simulink model "eVTOL_System"  (R2024b)
settings: Solver=FixedStepAuto  StartTime=0.0  StopTime=inf  RelTol=1e-3
undefined symbols (not defined in the file): airspeed, Battery, BCE12, BCE_Set_init, BMS_Controller_State, C, Cell10_P, Cell11_P, Cell12_P, Cell13_P, Cell14_P, Cell15_P, Cell16_P, Cell17_P, Cell18_P, Cell19_P, Cell1_N, Cell1_P, Cell20_P, Cell21_P, Cell22_P, Cell23_P, Cell24_P, Cell2_P, Cell3_P, Cell4_P, Cell5_P, Cell6_P, Cell7_P, Cell8_P, Cell9_P, Charging_State, CityMission, control, controlParams, ControlSampleTime, CriticalTiltAngle, currentFactor, CV_Gain, ddx, ddy, ddz, Device_01, Device_02, DiscIntNeverNeededParam, dx, dy, dz, Earth, env, F, F28379D_ADC_MaxCount, F28379D_ADC_Vmax, FixedWingMission, flightState, Foc_Ki_IxTcpu, Foc_Ki_S, Foc_Kp_I, Foc_Kp_S, fractalcoef ... (+68)
libraries: fl_lib x1115, nesl_utility x617, slrealtimeethercatlib x217, simulink x130, canmsglib x101, speedgoatlib_IO611_obsolete x91, slpidlib x49, mcbcontrolslib x44, slrealtimeutilitieslib x35, speedgoatlib_hdlCoder_IO3xx x31, dspstat3 x24, mcbpositiondecoderlib x12
(part 6 of 31)

== system eVTOL_System/Battery System/Battery/Battery Pack/100-Cell ==
  Ambient_Temperature : Inport
  Controlled Temperature Source : fl_lib/Thermal/Thermal Sources/Controlled Temperature Source
      settings: LibrarySourceBlock=|
      | BatteryPack_lib/CellModule1TC/Controlled
      | Temperature Source
  Delay : Delay
  Delay1 : Delay
  Delay2 : Delay
  Faults : Subsystem
  Faults1 : Subsystem
  Faults2 : Subsystem
  Module3 : BatteryModuleLibrary96v_lib/Module1  BatteryCapacityCell=100 A*hr  ExtrapolationMethodCell=simscape.enum.extrapolation.nearest  SOCBreakpointsCell=[0, .1, .25, .5, .75, .9, 1]  TemperatureBreakpointsCell=[278, 293, 313] K  OpenCircuitVoltageThermalCell=[3.49, 3.5, 3.51; 3.55, 3.57, 3.56; 3.62, 3.63, 3.64; 3.71, 3.71, 3.72; 3.91, 3.93, 3.94; 4.07, 4.08, 4.08; 4.19, 4.19, 4.19] V  VoltageRangeCell=[0, inf] V  ResistanceSOCBreakpointsCell=[0, .1, .25, .5, .75, .9, 1]  ResistanceTemperatureBreakpointsCell=[278, 293, 313] K  R0ThermalCell=[.00117, .00085, .0009; .0011, .00085, .0009; .00114, .00087, .00092; .00107, .00082, .00088; .00107, .00083, .00091; .00113, .00085, .00089; .00116, .00085, .00089] Ohm  BatteryThermalMassCell=1000 J/K  AmbientResistance=25 K/W  P=1  S=24  socCell_specify=off  socCell_priority=High  socCell=repmat(1, 24, 1)  socCell_nominal_specify=off  socCell_nominal_value=1  socCell_nominal_unit=1  numCycles_specify=off  numCycles_priority=High  numCycles=repmat(0, 24, 1)  numCycles_nominal_specify=off  numCycles_nominal_value=1  numCycles_nominal_unit=1  batteryVoltage_specify=off  batteryVoltage_priority=None  batteryVoltage=repmat(0, 24, 1) V  batteryVoltage_nominal_specify=off  batteryVoltage_nominal_value=1  batteryVoltage_nominal_unit=V  batteryCurrent_specify=off  batteryCurrent_priority=None  batteryCurrent=repmat(0, 24, 1) A  batteryCurrent_nominal_specify=off  batteryCurrent_nominal_value=1  batteryCurrent_nominal_unit=A  batteryTemperature_specify=off  batteryTemperature_priority=High  batteryTemperature=repmat(298.15, 24, 1) K  batteryTemperature_nominal_specify=off  batteryTemperature_nominal_value=1  batteryTemperature_nominal_unit=K  vParallelAssembly_specify=off  vParallelAssembly_priority=None  vParallelAssembly=repmat(0, 24, 1) V  vParallelAssembly_nominal_specify=off  vParallelAssembly_nominal_value=1  vParallelAssembly_nominal_unit=V  socParallelAssembly_specify=off  socParallelAssembly_priority=None  socParallelAssembly=repmat(1, 24, 1)  socParallelAssembly_nominal_specify=off  socParallelAssembly_nominal_value=1  socParallelAssembly_nominal_unit=1
      settings: InternalSimscapePortConfiguration="{\"Bottom\":[{\"id\":\"n\",\"label\":\"-\",\"type\":\"foundation.electrical.electrical\"}],\"Left\":[{\"id\":\"AmbH\",\"label\":\"AmbH\",\"type\":\"foundation.thermal.thermal\"}],\"Right\":[{\"id\":\"PositiveBus\",\"label\":\"+Bus\",\"type\":\"foundation.electrical.electrical\"},{\"id\":\"NegativeBus\",\"label\":\"-Bus\",\"type\":\"foundation.electrical.electrical\"}],\"Top\":[{\"id\":\"p\",\"label\":\"+\",\"type\":\"foundation.electrical.electrical\"}]}"
  Module4 : BatteryModuleLibrary150V_lib/Module1  BatteryCapacityCell=100 A*hr  ExtrapolationMethodCell=simscape.enum.extrapolation.nearest  SOCBreakpointsCell=[0, .1, .25, .5, .75, .9, 1]  TemperatureBreakpointsCell=[278, 293, 313] K  OpenCircuitVoltageThermalCell=[3.49, 3.5, 3.51; 3.55, 3.57, 3.56; 3.62, 3.63, 3.64; 3.71, 3.71, 3.72; 3.91, 3.93, 3.94; 4.07, 4.08, 4.08; 4.19, 4.19, 4.19] V  VoltageRangeCell=[0, inf] V  ResistanceSOCBreakpointsCell=[0, .1, .25, .5, .75, .9, 1]  ResistanceTemperatureBreakpointsCell=[278, 293, 313] K  R0ThermalCell=[.00117, .00085, .0009; .0011, .00085, .0009; .00114, .00087, .00092; .00107, .00082, .00088; .00107, .00083, .00091; .00113, .00085, .00089; .00116, .00085, .00089] Ohm  BatteryThermalMassCell=1000 J/K  AmbientResistance=25 K/W  P=1  S=38  socCell_specify=off  socCell_priority=High  socCell=repmat(1, 38, 1)  socCell_nominal_specify=off  socCell_nominal_value=1  socCell_nominal_unit=1  numCycles_specify=off  numCycles_priority=High  numCycles=repmat(0, 38, 1)  numCycles_nominal_specify=off  numCycles_nominal_value=1  numCycles_nominal_unit=1  batteryVoltage_specify=off  batteryVoltage_priority=None  batteryVoltage=repmat(0, 38, 1) V  batteryVoltage_nominal_specify=off  batteryVoltage_nominal_value=1  batteryVoltage_nominal_unit=V  batteryCurrent_specify=off  batteryCurrent_priority=None  batteryCurrent=repmat(0, 38, 1) A  batteryCurrent_nominal_specify=off  batteryCurrent_nominal_value=1  batteryCurrent_nominal_unit=A  batteryTemperature_specify=off  batteryTemperature_priority=High  batteryTemperature=repmat(298.15, 38, 1) K  batteryTemperature_nominal_specify=off  batteryTemperature_nominal_value=1  batteryTemperature_nominal_unit=K  vParallelAssembly_specify=off  vParallelAssembly_priority=None  vParallelAssembly=repmat(0, 38, 1) V  vParallelAssembly_nominal_specify=off  vParallelAssembly_nominal_value=1  vParallelAssembly_nominal_unit=V  socParallelAssembly_specify=off  socParallelAssembly_priority=None  socParallelAssembly=repmat(1, 38, 1)  socParallelAssembly_nominal_specify=off  socParallelAssembly_nominal_value=1  socParallelAssembly_nominal_unit=1
      settings: InternalSimscapePortConfiguration="{\"Bottom\":[{\"id\":\"n\",\"label\":\"-\",\"type\":\"foundation.electrical.electrical\"}],\"Left\":[{\"id\":\"AmbH\",\"label\":\"AmbH\",\"type\":\"foundation.thermal.thermal\"}],\"Right\":[{\"id\":\"PositiveBus\",\"label\":\"+Bus\",\"type\":\"foundation.electrical.electrical\"},{\"id\":\"NegativeBus\",\"label\":\"-Bus\",\"type\":\"foundation.electrical.electrical\"}],\"Top\":[{\"id\":\"p\",\"label\":\"+\",\"type\":\"foundation.electrical.electrical\"}]}"
  Module5 : BatteryModuleLibrary150V_lib/Module1  BatteryCapacityCell=100 A*hr  ExtrapolationMethodCell=simscape.enum.extrapolation.nearest  SOCBreakpointsCell=[0, .1, .25, .5, .75, .9, 1]  TemperatureBreakpointsCell=[278, 293, 313] K  OpenCircuitVoltageThermalCell=[3.49, 3.5, 3.51; 3.55, 3.57, 3.56; 3.62, 3.63, 3.64; 3.71, 3.71, 3.72; 3.91, 3.93, 3.94; 4.07, 4.08, 4.08; 4.19, 4.19, 4.19] V  VoltageRangeCell=[0, inf] V  ResistanceSOCBreakpointsCell=[0, .1, .25, .5, .75, .9, 1]  ResistanceTemperatureBreakpointsCell=[278, 293, 313] K  R0ThermalCell=[.00117, .00085, .0009; .0011, .00085, .0009; .00114, .00087, .00092; .00107, .00082, .00088; .00107, .00083, .00091; .00113, .00085, .00089; .00116, .00085, .00089] Ohm  BatteryThermalMassCell=1000 J/K  AmbientResistance=25 K/W  P=1  S=38  socCell_specify=off  socCell_priority=High  socCell=repmat(1, 38, 1)  socCell_nominal_specify=off  socCell_nominal_value=1  socCell_nominal_unit=1  numCycles_specify=off  numCycles_priority=High  numCycles=repmat(0, 38, 1)  numCycles_nominal_specify=off  numCycles_nominal_value=1  numCycles_nominal_unit=1  batteryVoltage_specify=off  batteryVoltage_priority=None  batteryVoltage=repmat(0, 38, 1) V  batteryVoltage_nominal_specify=off  batteryVoltage_nominal_value=1  batteryVoltage_nominal_unit=V  batteryCurrent_specify=off  batteryCurrent_priority=None  batteryCurrent=repmat(0, 38, 1) A  batteryCurrent_nominal_specify=off  batteryCurrent_nominal_value=1  batteryCurrent_nominal_unit=A  batteryTemperature_specify=off  batteryTemperature_priority=High  batteryTemperature=repmat(298.15, 38, 1) K  batteryTemperature_nominal_specify=off  batteryTemperature_nominal_value=1  batteryTemperature_nominal_unit=K  vParallelAssembly_specify=off  vParallelAssembly_priority=None  vParallelAssembly=repmat(0, 38, 1) V  vParallelAssembly_nominal_specify=off  vParallelAssembly_nominal_value=1  vParallelAssembly_nominal_unit=V  socParallelAssembly_specify=off  socParallelAssembly_priority=None  socParallelAssembly=repmat(1, 38, 1)  socParallelAssembly_nominal_specify=off  socParallelAssembly_nominal_value=1  socParallelAssembly_nominal_unit=1
      settings: InternalSimscapePortConfiguration="{\"Bottom\":[{\"id\":\"n\",\"label\":\"-\",\"type\":\"foundation.electrical.electrical\"}],\"Left\":[{\"id\":\"AmbH\",\"label\":\"AmbH\",\"type\":\"foundation.thermal.thermal\"}],\"Right\":[{\"id\":\"PositiveBus\",\"label\":\"+Bus\",\"type\":\"foundation.electrical.electrical\"},{\"id\":\"NegativeBus\",\"label\":\"-Bus\",\"type\":\"foundation.electrical.electrical\"}],\"Top\":[{\"id\":\"p\",\"label\":\"+\",\"type\":\"foundation.electrical.electrical\"}]}"
  Mux : Mux  Inputs=3
  Mux1 : Mux  Inputs=3
  Mux2 : Mux  Inputs=3
  PS-Simulink Converter{,1..2,5..6} (5 alike) : nesl_utility/PS-Simulink Converter  PhysicalDomain=network_engine_domain  SubClassName=ps_output  LeftPortType=input  RightPortType=output  PseudoPeriodic=off  Frequencies=[]  VectorFormat=inherit  Unit=inherit  AffineConversion=off
  Passive Balancing Interface : batt_lib/HIL/Passive Balancing Interface  balancingCircuitCount=24
      settings: InternalSimscapePortConfiguration="{\"Bottom\":[],\"Left\":[{\"id\":\"PositiveBus\",\"label\":\"+\",\"type\":\"foundation.electrical.electrical\"},{\"id\":\"NegativeBus\",\"label\":\"-\",\"type\":\"foundation.electrical.electrical\"}],\"Right\":[{\"id\":\"balancingCurrent\",\"label\":\"Ibat\",\"type\":\"input\"},{\"id\":\"balancingVoltage\",\"label\":\"Vbat\",\"type\":\"output\"}],\"Top\":[]}"
  Passive Balancing Interface1 : batt_lib/HIL/Passive Balancing Interface  balancingCircuitCount=38
      settings: InternalSimscapePortConfiguration="{\"Bottom\":[],\"Left\":[{\"id\":\"PositiveBus\",\"label\":\"+\",\"type\":\"foundation.electrical.electrical\"},{\"id\":\"NegativeBus\",\"label\":\"-\",\"type\":\"foundation.electrical.electrical\"}],\"Right\":[{\"id\":\"balancingCurrent\",\"label\":\"Ibat\",\"type\":\"input\"},{\"id\":\"balancingVoltage\",\"label\":\"Vbat\",\"type\":\"output\"}],\"Top\":[]}"
  Passive Balancing Interface2 : batt_lib/HIL/Passive Balancing Interface  balancingCircuitCount=38
      settings: InternalSimscapePortConfiguration="{\"Bottom\":[],\"Left\":[{\"id\":\"PositiveBus\",\"label\":\"+\",\"type\":\"foundation.electrical.electrical\"},{\"id\":\"NegativeBus\",\"label\":\"-\",\"type\":\"foundation.electrical.electrical\"}],\"Right\":[{\"id\":\"balancingCurrent\",\"label\":\"Ibat\",\"type\":\"input\"},{\"id\":\"balancingVoltage\",\"label\":\"Vbat\",\"type\":\"output\"}],\"Top\":[]}"
  Probe : SimscapeProbe  BoundBlock=16864  Variables={batteryTemperature, batteryVoltage, socParallelAssembly}
  Probe1 : SimscapeProbe  BoundBlock=17225  Variables={batteryTemperature, batteryVoltage, socParallelAssembly}
  Probe2 : SimscapeProbe  BoundBlock=17226  Variables={batteryTemperature, batteryVoltage, socParallelAssembly}
  Simulink-PS Converter{,1..3} (4 alike) : nesl_utility/Simulink-PS Converter  PhysicalDomain=network_engine_domain  SubClassName=ps_input  LeftPortType=input  RightPortType=output  PseudoPeriodic=off  Frequencies=[]  NoiseDistribution=none  NoiseParameters=[]  Unit=1  AffineConversion=off  FilteringAndDerivatives=provide  SimscapeFilterOrder=1  InputFilterTimeConstant=0.001  UdotUserProvided=0
      Simulink-PS Converter1 settings: LibrarySourceBlock=|
      | BatteryPack_lib/CellModule1TC/Simulink-PS
      | Converter1
  Terminator : Terminator
  Terminator1 : Terminator
  Terminator2 : Terminator
  Trigger_Faults : Subsystem
  Voltage Sensor : fl_lib/Electrical/Electrical Sensors/Voltage Sensor
  Voltage Sensor1 : fl_lib/Electrical/Electrical Sensors/Voltage Sensor
  Batt+ : PMIOPort  Side=Right
  Batt- : PMIOPort  Port=2  Side=Right
  Cells : PMIOPort  Port=3  Side=Right
  Cells1 : PMIOPort  Port=4  Side=Right
  Cells2 : PMIOPort  Port=5  Side=Right
  Cell_Voltages : Outport
  Cell_Temperatures : Outport  Port=2
  Cell_SOCs : Outport  Port=3
  tag scope: Cell_Voltages1=global, Cell_Voltages2=global, Pack_Voltage_24Cells=global, Pack_Voltage_76Cells=global
  wires:
  [Balancing_Currents] -> Delay/1
  Delay/1 -> Simulink-PS Converter/1
  Ambient_Temperature/1 -> Simulink-PS Converter1/1
  [Balancing_Currents1] -> Delay1/1
  Delay1/1 -> Simulink-PS Converter2/1
  [Balancing_Currents2] -> Delay2/1
  Delay2/1 -> Simulink-PS Converter3/1
  Mux1/1 -> Cell_Voltages/1
  Mux/1 -> Cell_Temperatures/1
  Mux2/1 -> Cell_SOCs/1
  Probe1/2 -> [Cell_Voltages1], [Vol2]
  Probe/1 -> [Temp1]
  Probe/2 -> [Vol1]
  Probe/3 -> [soc1]
  Probe1/1 -> [Temp2]
  Probe1/3 -> [soc2]
  Probe2/1 -> [Temp3]
  Probe2/2 -> [Cell_Voltages2], [Vol3]
  Probe2/3 -> [soc3]
  [Vol1] -> Mux1/1
  [Vol2] -> Mux1/2
  [Vol3] -> Mux1/3
  [Temp1] -> Mux/1
  [Temp2] -> Mux/2
  [Temp3] -> Mux/3
  [soc1] -> Mux2/1
  [soc2] -> Mux2/2
  [soc3] -> Mux2/3
  PS-Simulink Converter5/1 -> [Pack_Voltage_76Cells]
  PS-Simulink Converter6/1 -> [Pack_Voltage_24Cells]
  PS-Simulink Converter/1 -> Terminator/1
  Trigger_Faults/1(ShortCircuit) -> Faults/1(Short_Circuits), Faults2/1(Short_Circuits), Faults1/1(Short_Circuits)
  PS-Simulink Converter1/1 -> Terminator1/1
  PS-Simulink Converter2/1 -> Terminator2/1
  connections:
  Module3/LConn1 -- Module4/LConn1 -- Module5/LConn1 -- Controlled Temperature Source/LConn1
  Passive Balancing Interface/LConn1 -- Module3/RConn1 -- Faults/RConn1
  Passive Balancing Interface/RConn1 -- Simulink-PS Converter/RConn1
  PS-Simulink Converter/LConn1 -- Passive Balancing Interface/RConn2
  Passive Balancing Interface/LConn2 -- Module3/RConn2 -- Faults/RConn3
  Cells/RConn1 -- Faults/RConn2
  Simulink-PS Converter1/RConn1 -- Controlled Temperature Source/RConn1
  Module5/LConn2 -- Voltage Sensor1/LConn1 -- Voltage Sensor/RConn2 -- Module3/RConn3
  Batt-/RConn1 -- Voltage Sensor1/RConn2 -- Module4/RConn3
  Module4/LConn2 -- Module5/RConn3
  Faults1/RConn3 -- Module5/RConn2 -- Passive Balancing Interface1/LConn2
  Faults1/RConn1 -- Module5/RConn1 -- Passive Balancing Interface1/LConn1
  Passive Balancing Interface1/RConn1 -- Simulink-PS Converter2/RConn1
  Cells1/RConn1 -- Faults1/RConn2
  PS-Simulink Converter1/LConn1 -- Passive Balancing Interface1/RConn2
  Passive Balancing Interface2/LConn2 -- Faults2/RConn3 -- Module4/RConn2
  Passive Balancing Interface2/LConn1 -- Faults2/RConn1 -- Module4/RConn1
  Passive Balancing Interface2/RConn1 -- Simulink-PS Converter3/RConn1
  Faults2/RConn2 -- Cells2/RConn1
  PS-Simulink Converter2/LConn1 -- Passive Balancing Interface2/RConn2
  PS-Simulink Converter5/LConn1 -- Voltage Sensor1/RConn1
  PS-Simulink Converter6/LConn1 -- Voltage Sensor/RConn1
  Batt+/RConn1 -- Voltage Sensor/LConn1 -- Module3/LConn2

== system eVTOL_System/Battery System/Battery/HW Interface/BCE - HIL ==
  Sensor_Values_Sim : Inport
  Add : Sum  Inputs=+
  Add1 : Sum  Inputs=+
  Add2 : Sum  Inputs=+
  Battery Cell Emulator : Subsystem
  Bus Creator : BusCreator  Inputs=6
  Data Type Conversion : DataTypeConversion  SaturateOnIntegerOverflow=off  RndMeth=Floor
  Selector1 : Subsystem
  Shunt Emulator : Subsystem
  Temperature Emulator : Subsystem
  Cells_IN : PMIOPort  Side=Left
  Cells_OUT : PMIOPort  Port=2  Side=Right
  Sensor_Values_Real : Outport
  tag scope: Balancing_Currents=global
  wires:
  Sensor_Values_Sim/1 -> Battery Cell Emulator/1(Sensor_Values_Sim), Shunt Emulator/1(Sensor_Values_Sim), Temperature Emulator/1(Sensor_Values_Sim)
  Battery Cell Emulator/2(Cell_Voltages) -> Add1/1, Selector1/1(24Cells)
  Temperature Emulator/1(Cell_Temperatures) -> Bus Creator/2  "Cell_Temperatures"
  Add/1 -> Bus Creator/3  "Pack_Voltage"
  Bus Creator/1 -> Sensor_Values_Real/1
  Battery Cell Emulator/1(Current_Values) -> Data Type Conversion/1
  Data Type Conversion/1 -> [Balancing_Currents]
  Selector1/1(100Cells) -> Bus Creator/1, Add/1  "Cell_Voltages"
  Battery Cell Emulator/3(OtherVoltages) -> Add2/1, Selector1/2(76Cells)
  Add1/1 -> Bus Creator/4  "Pack_Voltage1"
  Add2/1 -> Bus Creator/5  "Pack_Voltage2"
  Shunt Emulator/1(Pack_Current) -> Bus Creator/6  "Pack_Current"
  connections:
  Cells_OUT/RConn1 -- Cells_IN/RConn1

== system eVTOL_System/Battery System/Battery/HW Interface/MIL ==
  Sensor_Values_Sim : Inport
  Cells_IN : PMIOPort  Side=Left
  Cells_OUT : PMIOPort  Port=2  Side=Right
  Sensor_Values_Real : Outport
  wires:
  Sensor_Values_Sim/1 -> Sensor_Values_Real/1
  connections:
  Cells_IN/RConn1 -- Cells_OUT/RConn1

== system eVTOL_System/Battery System/Battery/Override/Celsius_to_Kelvin ==
  C : Inport
  Add : Sum
  Constant4 : Constant  Value=273.15
  K : Outport
  wires:
  Constant4/1 -> Add/2
  C/1 -> Add/1
  Add/1 -> K/1

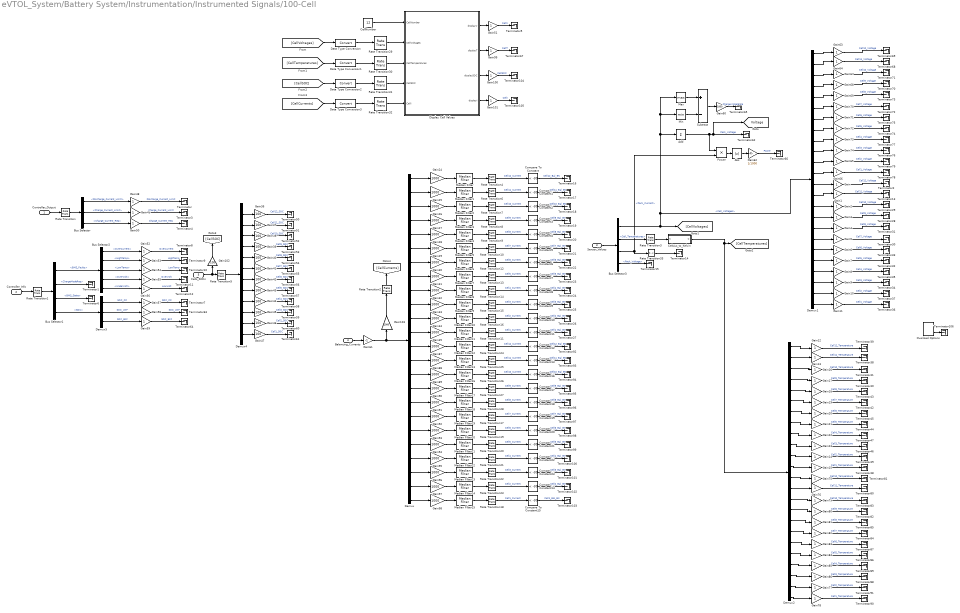
== system eVTOL_System/Battery System/Instrumentation/Instrumented Signals/100-Cell ==
  Controller_Output : Inport
  Controller_Info : Inport  Port=2
  Sensor_Values : Inport  Port=3
  Balancing_Currents : Inport  Port=4
  Cells_SOCs : Inport  Port=5
  Abs : Abs  SaturateOnIntegerOverflow=off
  Add : Sum  Inputs=+
  Bus Selector : BusSelector  OutputSignals=Discharge_Current_Limit,Charge_Current_Limit,Charge_Current_Req
  Bus Selector1 : BusSelector  OutputSignals=BMS_Faults,ChargeModeReq,BMS_State,SOC
  Bus Selector2 : BusSelector  OutputSignals=OverCurrent,HighTemp,LowTemp,OverVolt,UnderVolt
  Bus Selector3 : BusSelector  OutputSignals=Cell_Voltages,Cell_Temperatures,Pack_Current,Pack_Voltage
  CellNumber : Constant  Value=12
  Celsius_to_Kelvin : Subsystem
  Compare To Constant{,1..23} (24 alike) : simulink/Logic and Bit Operations/Compare To Constant  relop=<  const=-30  OutDataTypeStr=boolean
  Data Type Conversion{,1..3} (4 alike) : DataTypeConversion  SaturateOnIntegerOverflow=off  RndMeth=Floor
  Demux : Demux  Outputs=24
  Demux1 : Demux  Outputs=24
  Demux2 : Demux  Outputs=24
  Demux4 : Demux  Outputs=12
  Demux5 : Demux  Outputs=3
  Display Cell Values : MATLAB Function  TreatAsAtomicUnit=on
  Gain{,1..23,48..59,63..86,99..101} (63 alike) : Gain
  Gain{36..47,102} (13 alike) : Gain  Gain=100
  Gain{24..35,60,87..98,103} (26 alike) : Gain  Gain=1000
  Gain61 : Gain  Gain=-1
  Gain62 : Gain  Gain=1/1000
  Max : MinMax  Function=max
  Median Filter{,1..23} (24 alike) : dspstat3/Median Filter  WindowLength=7  SimulateUsing=Code generation
  Min : MinMax
  Overload Options : slrealtimetgmanagement/Overload Options  startupDur=1  startupDurSrc=Tunable Parameter  maxOverload=100000000  maxOverloadSrc=Tunable Parameter  TETFlag=on
  Power : Product
  Rate Transition{,1..28} (29 alike) : RateTransition  OutPortSampleTime=0.1
  Rate Transition{29..32} (4 alike) : RateTransition
  Rate Transition33 : RateTransition  OutPortSampleTime=0.01
  Subtract : Sum  Inputs=+-
  Terminator{,1..106} (107 alike) : Terminator
  tag scope: Voltage=global
  wires:
  Controller_Output/1 -> Rate Transition/1
  Controller_Info/1 -> Rate Transition1/1
  Sensor_Values/1 -> Bus Selector3/1
  Bus Selector/1 -> Gain48/1  "<Discharge_Current_Limit>"
  Bus Selector/2 -> Gain49/1  "<Charge_Current_Limit>"
  Bus Selector/3 -> Gain50/1  "<Charge_Current_Req>"
  Rate Transition/1 -> Bus Selector/1
  Bus Selector1/2 -> Terminator1/1  "<ChargeModeReq>"
  Bus Selector1/3 -> Terminator6/1  "<BMS_State>"
  Bus Selector1/4 -> Demux5/1  "<SOC>"
  Bus Selector2/1 -> Gain52/1  "<OverCurrent>"
  Bus Selector2/2 -> Gain53/1  "<HighTemp>"
  Bus Selector2/3 -> Gain54/1  "<LowTemp>"
  Bus Selector2/4 -> Gain55/1  "<OverVolt>"
  Bus Selector2/5 -> Gain56/1  "<UnderVolt>"
  Rate Transition1/1 -> Bus Selector1/1
  Bus Selector3/1 -> [CellVoltages], Demux1/1, Add/1, Min/1, Max/1  "<Cell_Voltages>"
  Bus Selector3/2 -> Rate Transition3/1  "<Cell_Temperatures>"
  Bus Selector3/3 -> Power/2, Rate Transition33/1  "<Pack_Current>"
  Bus Selector3/4 -> Terminator15/1  "<Pack_Voltage>"
  Demux/1 -> Gain24/1
  Demux/2 -> Gain25/1
  Demux/3 -> Gain26/1
  Demux/6 -> Gain29/1
  Demux/5 -> Gain28/1
  Demux/4 -> Gain27/1
  Demux/9 -> Gain32/1
  Demux/11 -> Gain34/1
  Demux/7 -> Gain30/1
  Demux/8 -> Gain31/1
  Demux/10 -> Gain33/1
  Demux/12 -> Gain35/1
  Balancing_Currents/1 -> Gain61/1
  Gain/1 -> Terminator2/1  "Cell12_Voltage"
  Gain1/1 -> Terminator13/1  "Cell11_Voltage"
  Gain2/1 -> Terminator29/1  "Cell10_Voltage"
  Gain3/1 -> Terminator28/1  "Cell9_Voltage"
  Gain4/1 -> Terminator31/1  "Cell8_Voltage"
  Gain5/1 -> Terminator30/1  "Cell7_Voltage"
  Gain6/1 -> Terminator33/1  "Cell6_Voltage"
  Gain7/1 -> Terminator32/1  "Cell5_Voltage"
  Gain8/1 -> Terminator35/1  "Cell4_Voltage"
  Gain9/1 -> Terminator34/1  "Cell3_Voltage"
  Gain10/1 -> Terminator37/1  "Cell2_Voltage"
  Gain11/1 -> Terminator36/1  "Cell1_Voltage"
  Gain22/1 -> Terminator47/1  "Cell4_Temperature"
  Gain19/1 -> Terminator42/1  "Cell7_Temperature"
  Gain17/1 -> Terminator40/1  "Cell9_Temperature"
  Gain13/1 -> Terminator38/1  "Cell11_Temperature"
  Demux2/10 -> Gain23/1
  Demux2/12 -> Gain15/1
  Demux2/11 -> Gain14/1
  Demux2/9 -> Gain22/1
  Demux2/2 -> Gain13/1
  Gain14/1 -> Terminator49/1  "Cell2_Temperature"
  Demux2/3 -> Gain16/1
  Demux2/4 -> Gain17/1
  Demux2/1 -> Gain12/1
  Gain20/1 -> Terminator45/1  "Cell6_Temperature"
  Gain12/1 -> Terminator39/1  "Cell12_Temperature"
  Gain16/1 -> Terminator41/1  "Cell10_Temperature"
  Demux2/7 -> Gain20/1
  Demux2/6 -> Gain19/1
  Demux2/5 -> Gain18/1
  Gain21/1 -> Terminator44/1  "Cell5_Temperature"
  Rate Transition3/1 -> Celsius_to_Kelvin/1(K)
  Demux2/8 -> Gain21/1
  Gain18/1 -> Terminator43/1  "Cell8_Temperature"
  Gain15/1 -> Terminator48/1  "Cell1_Temperature"
  Gain23/1 -> Terminator46/1  "Cell3_Temperature"
  Celsius_to_Kelvin/1(C) -> [CellTemperatures], Demux2/1
  Rate Transition6/1 -> Compare To Constant1/1  "Cell11_Current"
  Rate Transition4/1 -> Compare To Constant/1  "Cell12_Current"
  Rate Transition8/1 -> Compare To Constant3/1  "Cell9_Current"
  Rate Transition7/1 -> Compare To Constant2/1  "Cell10_Current"
  Compare To Constant/1 -> Terminator16/1  "Cell12_Bal_EN"
  Compare To Constant1/1 -> Terminator17/1  "Cell11_Bal_EN"
  Compare To Constant3/1 -> Terminator19/1  "Cell9_Bal_EN"
  Compare To Constant2/1 -> Terminator18/1  "Cell10_Bal_EN"
  Compare To Constant5/1 -> Terminator21/1  "Cell7_Bal_EN"
  Compare To Constant4/1 -> Terminator20/1  "Cell8_Bal_EN"
  Rate Transition10/1 -> Compare To Constant5/1  "Cell7_Current"
  Rate Transition12/1 -> Compare To Constant6/1  "Cell6_Current"
  Compare To Constant6/1 -> Terminator22/1  "Cell6_Bal_EN"
  Rate Transition9/1 -> Compare To Constant4/1  "Cell8_Current"
  Rate Transition13/1 -> Compare To Constant7/1  "Cell5_Current"
  Compare To Constant7/1 -> Terminator23/1  "Cell5_Bal_EN"
  Compare To Constant9/1 -> Terminator25/1  "Cell3_Bal_EN"
  Compare To Constant8/1 -> Terminator24/1  "Cell4_Bal_EN"
  Rate Transition15/1 -> Compare To Constant9/1  "Cell3_Current"
  Rate Transition16/1 -> Compare To Constant10/1  "Cell2_Current"
  Compare To Constant10/1 -> Terminator26/1  "Cell2_Bal_EN"
  Rate Transition14/1 -> Compare To Constant8/1  "Cell4_Current"
  Rate Transition11/1 -> Compare To Constant11/1  "Cell1_Current"
  Compare To Constant11/1 -> Terminator27/1  "Cell1_Bal_EN"
  Cells_SOCs/1 -> Gain102/1, Rate Transition5/1
  Demux4/1 -> Gain36/1
  Demux4/2 -> Gain37/1
  Demux4/3 -> Gain38/1
  Demux4/4 -> Gain39/1
  Demux4/5 -> Gain40/1
  Demux4/6 -> Gain41/1
  Demux4/12 -> Gain47/1
  Demux4/11 -> Gain46/1
  Demux4/10 -> Gain45/1
  Demux4/9 -> Gain44/1
  Demux4/7 -> Gain42/1
  Demux4/8 -> Gain43/1
  Gain36/1 -> Terminator50/1  "Cell12_SOC"
  Gain37/1 -> Terminator51/1  "Cell11_SOC"
  Gain38/1 -> Terminator52/1  "Cell10_SOC"
  Gain39/1 -> Terminator53/1  "Cell9_SOC"
  Gain40/1 -> Terminator54/1  "Cell8_SOC"
  Gain41/1 -> Terminator55/1  "Cell7_SOC"
  Gain42/1 -> Terminator56/1  "Cell6_SOC"
  Gain43/1 -> Terminator57/1  "Cell5_SOC"
  Gain44/1 -> Terminator58/1  "Cell4_SOC"
  Gain45/1 -> Terminator59/1  "Cell3_SOC"
  Gain46/1 -> Terminator60/1  "Cell2_SOC"
  Gain47/1 -> Terminator61/1  "Cell1_SOC"
  Rate Transition5/1 -> Demux4/1
  Demux5/1 -> Gain57/1  "SOC_CC"
  Demux5/2 -> Gain58/1  "SOC_UKF"
  Demux5/3 -> Gain59/1  "SOC_EKF"
  Max/1 -> Subtract/1
  Min/1 -> Subtract/2
  Subtract/1 -> Gain60/1
  Gain48/1 -> Terminator/1  "Discharge_Current_Limit"
  Gain49/1 -> Terminator3/1  "Charge_Current_Limit"
  Gain50/1 -> Terminator4/1  "Charge_Current_Req"
  Gain52/1 -> Terminator8/1  "Overcurrent"
  Gain53/1 -> Terminator9/1  "HighTemp"
  Gain54/1 -> Terminator10/1  "LowTemp"
  Gain55/1 -> Terminator11/1  "OverVolt"
  Gain56/1 -> Terminator12/1  "LowVolt"
  Gain57/1 -> Terminator7/1  "SOC_CC"
  Gain59/1 -> Terminator64/1  "SOC_EKF"
  Bus Selector1/1 -> Bus Selector2/1  "<BMS_Faults>"
  Gain58/1 -> Terminator63/1  "SOC_UKF"
  Gain24/1 -> Median Filter/1
  Gain25/1 -> Median Filter1/1
  Gain26/1 -> Median Filter2/1
  Gain27/1 -> Median Filter3/1
  Gain28/1 -> Median Filter4/1
  Gain29/1 -> Median Filter5/1
  Gain32/1 -> Median Filter8/1
  Gain35/1 -> Median Filter11/1
  Gain30/1 -> Median Filter6/1
  Gain33/1 -> Median Filter9/1
  Gain34/1 -> Median Filter10/1
  Gain31/1 -> Median Filter7/1
  Gain60/1 -> Terminator65/1  "Charge Imbalance"
  Median Filter/1 -> Rate Transition4/1
  Median Filter1/1 -> Rate Transition6/1
  Median Filter2/1 -> Rate Transition7/1
  Median Filter3/1 -> Rate Transition8/1
  Median Filter4/1 -> Rate Transition9/1
  Median Filter5/1 -> Rate Transition10/1
  Median Filter6/1 -> Rate Transition12/1
  Median Filter7/1 -> Rate Transition13/1
  Median Filter8/1 -> Rate Transition14/1
  Median Filter9/1 -> Rate Transition15/1
  Median Filter10/1 -> Rate Transition16/1
  Median Filter11/1 -> Rate Transition11/1
  Add/1 -> Power/1, [Voltage], Terminator62/1  "Pack_Voltage"
  Power/1 -> Abs/1
  Abs/1 -> Gain62/1
  Gain64/1 -> Terminator68/1  "Cell11_Voltage"
  Gain65/1 -> Terminator79/1  "Cell2_Voltage"
  Gain66/1 -> Terminator78/1  "Cell1_Voltage"
  Gain73/1 -> Terminator77/1  "Cell4_Voltage"
  Gain74/1 -> Terminator76/1  "Cell3_Voltage"
  Gain72/1 -> Terminator74/1  "Cell5_Voltage"
  Gain69/1 -> Terminator73/1  "Cell8_Voltage"
  Gain67/1 -> Terminator71/1  "Cell10_Voltage"
  Gain71/1 -> Terminator75/1  "Cell6_Voltage"
  Gain70/1 -> Terminator72/1  "Cell7_Voltage"
  Gain63/1 -> Terminator69/1  "Cell12_Voltage"
  Gain68/1 -> Terminator70/1  "Cell9_Voltage"
  Demux1/13 -> Gain/1
  Demux1/15 -> Gain2/1
  Demux1/16 -> Gain3/1
  Demux1/17 -> Gain4/1
  Demux1/18 -> Gain5/1
  Demux1/19 -> Gain6/1
  Demux1/20 -> Gain7/1
  Demux1/21 -> Gain8/1
  Demux1/22 -> Gain9/1
  Demux1/23 -> Gain10/1
  Demux1/24 -> Gain11/1
  Demux1/1 -> Gain63/1
  Demux1/3 -> Gain67/1
  Demux1/4 -> Gain68/1
  Demux1/5 -> Gain69/1
  Demux1/6 -> Gain70/1
  Demux1/7 -> Gain71/1
  Demux1/8 -> Gain72/1
  Demux1/9 -> Gain73/1
  Demux1/10 -> Gain74/1
  Demux1/11 -> Gain65/1
  Demux1/12 -> Gain66/1
  Demux1/14 -> Gain1/1
  Demux1/2 -> Gain64/1
  Gain80/1 -> Terminator82/1  "Cell9_Temperature"
  Gain77/1 -> Terminator91/1  "Cell2_Temperature"
  Demux2/23 -> Gain77/1
  Demux2/24 -> Gain78/1
  Gain81/1 -> Terminator85/1  "Cell8_Temperature"
  Demux2/15 -> Gain79/1
  Demux2/21 -> Gain85/1
  Gain76/1 -> Terminator80/1  "Cell11_Temperature"
  Demux2/14 -> Gain76/1
  Demux2/19 -> Gain83/1
  Gain84/1 -> Terminator86/1  "Cell5_Temperature"
  Demux2/22 -> Gain86/1
  Demux2/20 -> Gain84/1
  Gain78/1 -> Terminator90/1  "Cell1_Temperature"
  Gain75/1 -> Terminator81/1  "Cell12_Temperature"
  Demux2/13 -> Gain75/1
  Gain79/1 -> Terminator83/1  "Cell10_Temperature"
  Demux2/16 -> Gain80/1
  Gain83/1 -> Terminator87/1  "Cell6_Temperature"
  Gain86/1 -> Terminator88/1  "Cell3_Temperature"
  Gain85/1 -> Terminator89/1  "Cell4_Temperature"
  Demux2/18 -> Gain82/1
  Gain82/1 -> Terminator84/1  "Cell7_Temperature"
  Demux2/17 -> Gain81/1
  Gain89/1 -> Median Filter16/1
  Rate Transition18/1 -> Compare To Constant15/1  "Cell1_Current"
  Gain98/1 -> Median Filter15/1
  Median Filter13/1 -> Rate Transition25/1
  Median Filter21/1 -> Rate Transition20/1
  Median Filter18/1 -> Rate Transition28/1
  Median Filter19/1 -> Rate Transition17/1
  Rate Transition25/1 -> Compare To Constant13/1  "Cell11_Current"
  Median Filter16/1 -> Rate Transition26/1
  Gain95/1 -> Median Filter22/1
  Compare To Constant21/1 -> Terminator99/1  "Cell5_Bal_EN"
  Demux/21 -> Gain95/1
  Gain92/1 -> Median Filter19/1
  Gain93/1 -> Median Filter20/1
  Compare To Constant19/1 -> Terminator97/1  "Cell7_Bal_EN"
  Gain96/1 -> Median Filter23/1
  Rate Transition20/1 -> Compare To Constant21/1  "Cell5_Current"
  Median Filter17/1 -> Rate Transition27/1
  Median Filter22/1 -> Rate Transition21/1
  Demux/24 -> Gain98/1
  Demux/15 -> Gain89/1
  Median Filter12/1 -> Rate Transition24/1
  Demux/14 -> Gain88/1
  Median Filter14/1 -> Rate Transition23/1
  Demux/23 -> Gain97/1
  Gain94/1 -> Median Filter21/1
  Demux/13 -> Gain87/1
  Demux/22 -> Gain96/1
  Rate Transition22/1 -> Compare To Constant23/1  "Cell3_Current"
  Compare To Constant17/1 -> Terminator95/1  "Cell9_Bal_EN"
  Compare To Constant18/1 -> Terminator96/1  "Cell8_Bal_EN"
  Compare To Constant23/1 -> Terminator101/1  "Cell3_Bal_EN"
  Compare To Constant15/1 -> Terminator103/1  "Cell1_Bal_EN"
  Rate Transition28/1 -> Compare To Constant18/1  "Cell8_Current"
  Compare To Constant22/1 -> Terminator100/1  "Cell4_Bal_EN"
  Demux/17 -> Gain91/1
  Demux/20 -> Gain94/1
  Median Filter15/1 -> Rate Transition18/1
  Rate Transition23/1 -> Compare To Constant14/1  "Cell2_Current"
  Compare To Constant14/1 -> Terminator102/1  "Cell2_Bal_EN"
  Rate Transition19/1 -> Compare To Constant20/1  "Cell6_Current"
  Gain88/1 -> Median Filter13/1
  Compare To Constant13/1 -> Terminator93/1  "Cell11_Bal_EN"
  Gain97/1 -> Median Filter14/1
  Gain90/1 -> Median Filter17/1
  Compare To Constant16/1 -> Terminator94/1  "Cell10_Bal_EN"
  Gain91/1 -> Median Filter18/1
  Compare To Constant20/1 -> Terminator98/1  "Cell6_Bal_EN"
  Compare To Constant12/1 -> Terminator92/1  "Cell12_Bal_EN"
  Rate Transition24/1 -> Compare To Constant12/1  "Cell12_Current"
  Median Filter23/1 -> Rate Transition22/1
  Median Filter20/1 -> Rate Transition19/1
  Rate Transition27/1 -> Compare To Constant17/1  "Cell9_Current"
  Demux/16 -> Gain90/1
  Rate Transition17/1 -> Compare To Constant19/1  "Cell7_Current"
  Demux/18 -> Gain92/1
  Rate Transition26/1 -> Compare To Constant16/1  "Cell10_Current"
  Rate Transition21/1 -> Compare To Constant22/1  "Cell4_Current"
  Demux/19 -> Gain93/1
  Gain87/1 -> Median Filter12/1
  Gain62/1 -> Terminator66/1  "Power"
  Gain61/1 -> Demux/1, Gain103/1
  [CellVoltages] -> Data Type Conversion/1
  [CellTemperatures] -> Data Type Conversion1/1
  CellNumber/1 -> Display Cell Values/1(CellNumber)
  [CellSOC] -> Data Type Conversion2/1
  [CellCurrents] -> Data Type Conversion3/1
  Display Cell Values/1(displayV) -> Gain51/1
  Display Cell Values/2(displayT) -> Gain99/1
  Display Cell Values/3(displaySOC) -> Gain100/1
  Display Cell Values/4(displayI) -> Gain101/1
  Gain51/1 -> Terminator5/1  "CellV"
  Gain99/1 -> Terminator67/1  "CellT"
  Gain100/1 -> Terminator104/1  "CellSOC"
  Gain101/1 -> Terminator105/1  "CellI"
  Gain102/1 -> [CellSOC]
  Data Type Conversion/1 -> Rate Transition29/1
  Data Type Conversion1/1 -> Rate Transition30/1
  Data Type Conversion2/1 -> Rate Transition31/1
  Data Type Conversion3/1 -> Rate Transition32/1
  Rate Transition2/1 -> [CellCurrents]
  Gain103/1 -> Rate Transition2/1
  Overload Options/2 -> Terminator106/1
  Rate Transition29/1 -> Display Cell Values/2(CellVoltages)
  Rate Transition30/1 -> Display Cell Values/3(CellTemperatures)
  Rate Transition31/1 -> Display Cell Values/4(CellSOC)
  Rate Transition32/1 -> Display Cell Values/5(CellI)
  Rate Transition33/1 -> Terminator14/1

== system eVTOL_System/Dynamics/Force and Moments/Aerodynamic Forces/Compute Air Data ==
  Vb : Inport  PortDimensions=3
  Rho : Inport  Port=2
  Bus Creator : BusCreator  Inputs=4
  Dynamic Pressure : aerolibasang/Dynamic Pressure
  "Incidence, Sideslip, & Airspeed" : aerolibasang/Incidence, Sideslip, & Airspeed
  Saturation : Saturate  UpperLimit=14*pi/180  LowerLimit=-14*pi/180
  Scope : Scope
  AirData : Outport  VectorParamsAs1DForOutWhenUnconnected=off
  wires:
  Bus Creator/1 -> Scope/1, AirData/1
  "Incidence, Sideslip, & Airspeed"/1 -> Bus Creator/1  "alpha"
  Rho/1 -> Dynamic Pressure/2
  "Incidence, Sideslip, & Airspeed"/3 -> Bus Creator/3  "airspeed"
  Dynamic Pressure/1 -> Bus Creator/4  "q"
  Vb/1 -> "Incidence, Sideslip, & Airspeed"/1, Dynamic Pressure/1
  "Incidence, Sideslip, & Airspeed"/2 -> Saturation/1  "beta"
  Saturation/1 -> Bus Creator/2  "beta"

== system eVTOL_System/Dynamics/Force and Moments/Aerodynamic Forces/Compute Body Frame Forces and Moments ==
  AirData : Inport
  CtrlSurfaces : Inport  Port=2
  p,q,r : Inport  Port=3
  Bus Selector : BusSelector  OutputSignals=alpha,beta
  Mux : Mux  Inputs=2
  Rotate FM to body frame : Subsystem
  Wind frame F& M : Subsystem
  F_b : Outport  Unit=kg*m/s^2  VectorParamsAs1DForOutWhenUnconnected=off
  M_b : Outport  Port=2  Unit=kg*m/s  VectorParamsAs1DForOutWhenUnconnected=off
  wires:
  Mux/1 -> Rotate FM to body frame/2(alpha_beta)
  Bus Selector/2 -> Mux/2  "<beta>"
  Bus Selector/1 -> Mux/1  "<alpha>"
  Wind frame F& M/1(FM_w) -> Rotate FM to body frame/1(FM_w)  "FM_W"
  p,q,r/1 -> Wind frame F& M/3(p,q,r)
  Rotate FM to body frame/2(M_b) -> M_b/1
  Rotate FM to body frame/1(F_b) -> F_b/1
  CtrlSurfaces/1 -> Wind frame F& M/2(CtrlSurfaces)
  AirData/1 -> Wind frame F& M/1(Airdata), Bus Selector/1

== system eVTOL_System/Dynamics/Force and Moments/Aerodynamic Forces/Rotate Vw ==
  Vw : Inport
  Euler : Inport  Port=2
  RL2B : mbdriLib/Coordinates/RL2B  SystemSampleTime=-1  VariantActivationTime=update diagram  AllowFlexibleInterface=on  Latency=0  AutoFrameSizeCalculation=off
  RL2B * Vw : Product  Multiplication=Matrix(*)  InputSameDT=on  SaturateOnIntegerOverflow=on  OutDataTypeStr=Inherit: Same as first input
  Vb : Outport  Unit=m/s  VectorParamsAs1DForOutWhenUnconnected=off
  wires:
  RL2B * Vw/1 -> Vb/1
  Vw/1 -> RL2B * Vw/2
  RL2B/1 -> RL2B * Vw/1
  Euler/1 -> RL2B/1

== system eVTOL_System/Dynamics/Force and Moments/Propulsion/Tilt Servo Dynamics ==
  TiltA : Inport
  TiltB : Inport  Port=2
  Gain2 : Gain  Gain=pi/2
  Gain3 : Gain  Gain=pi/2
  IC : InitialCondition  Value=tiltIni
  IC1 : InitialCondition  Value=tiltIni
  Servo Dynamics : TransferFcn  Denominator=[0.1 1]
  Servo Dynamics1 : TransferFcn  Denominator=[0.1 1]
  Tilt1 : Outport
  Tilt2 : Outport  Port=2
  wires:
  Gain2/1 -> Servo Dynamics/1
  TiltB/1 -> Gain3/1
  Servo Dynamics/1 -> IC1/1
  Servo Dynamics1/1 -> IC/1
  IC/1 -> Tilt2/1  "Tilt2"
  IC1/1 -> Tilt1/1  "Tilt1"
  Gain3/1 -> Servo Dynamics1/1
  TiltA/1 -> Gain2/1

== system eVTOL_System/Dynamics/Force and Moments/Weather Model/Simple Model ==
  AirData : Inport
  Xe : Inport  Port=2
  Euler : Inport  Port=3
  Constant : Constant  Value=[ 0 0 0]
      settings: AttributesFormatString=%<Value>
  Constant1 : Constant  Value=uavParam.aero.rho
  Terminator : Terminator
  Terminator1 : Terminator
  Terminator3 : Terminator
  Wind_e : Outport  Unit=m/s  VectorParamsAs1DForOutWhenUnconnected=off
  " Rho" : Outport  Port=2  VectorParamsAs1DForOutWhenUnconnected=off
  wires:
  AirData/1 -> Terminator/1
  Constant/1 -> Wind_e/1
  Euler/1 -> Terminator1/1
  Xe/1 -> Terminator3/1
  Constant1/1 -> " Rho"/1

== system eVTOL_System/Dynamics/Force and Moments/Weather Model/Weather Model ==
  AirData : Inport
  Xe : Inport  Port=2
  Euler : Inport  Port=3
  Add : Sum  Inputs=2
  Bus Selector : BusSelector  OutputSignals=airspeed
  Constant1 : Constant  Value=uavParam.aero.rho
  Dryden Wind Turbulence Model (Discrete (+q -r)) : aerolibwind2/Dryden Wind Turbulence Model  (Continuous (+q -r))  units=Metric (MKS)  spec=MIL-F-8785C  model=Discrete Dryden (+q -r)  W20=env.windBase/4  Wdeg=env.windDirTurb  TurbProb=10^-2 - Light  L_high=533.4  Wingspan=uavParam.geom.b  ts=0.005  Seed=[23341 23342 23343 23344]  T_on=on
  Gain : Gain  Gain=-1
      settings: AttributesFormatString=Z to Alt
  Get Z : Selector  InputPortWidth=3  IndexOptions=Index vector (dialog)  Indices=[3]  OutputSizes=[(-2)]
  Horizontal Wind Model : aerolibwind2/Horizontal Wind Model  units=Metric (MKS)  Vw_source=Internal  Vwind=env.windBase  W_source=Internal  Wdeg=env.windDirHor
  RL2B : mbdriLib/Coordinates/RL2B  SystemSampleTime=-1  VariantActivationTime=update diagram  AllowFlexibleInterface=on  Latency=0  AutoFrameSizeCalculation=off
  Reduce Z Wind : Gain  Gain=[1 1 0.1]
      settings: AttributesFormatString=%<Gain>
  Rotate to E Frame : Product  Multiplication=Matrix(*)
  Terminator : Terminator
  Transfer Fcn : TransferFcn  Denominator=[.01 1]
  Transfer Fcn1 : TransferFcn  Denominator=[.01 1]
  Transpose : Math  Operator=transpose  SignedPower=on
  Wind_e : Outport  Unit=m/s  VectorParamsAs1DForOutWhenUnconnected=off
  Rho : Outport  Port=2  VectorParamsAs1DForOutWhenUnconnected=off
  wires:
  Bus Selector/1 -> Transfer Fcn1/1  "<airspeed>"
  AirData/1 -> Bus Selector/1
  Transfer Fcn/1 -> Gain/1
  Dryden Wind Turbulence Model (Discrete (+q -r))/2 -> Terminator/1
  Reduce Z Wind/1 -> Add/1
  Dryden Wind Turbulence Model (Discrete (+q -r))/1 -> Reduce Z Wind/1
  Rotate to E Frame/1 -> Wind_e/1
  Transpose/1 -> Rotate to E Frame/1
  Horizontal Wind Model/1 -> Add/2
  Transfer Fcn1/1 -> Dryden Wind Turbulence Model (Discrete (+q -r))/2
  Add/1 -> Rotate to E Frame/2
  RL2B/1 -> Dryden Wind Turbulence Model (Discrete (+q -r))/3, Horizontal Wind Model/1, Transpose/1  "RECEF2B"
  Euler/1 -> RL2B/1
  Get Z/1 -> Transfer Fcn/1
  Xe/1 -> Get Z/1
  Gain/1 -> Dryden Wind Turbulence Model (Discrete (+q -r))/1
  Constant1/1 -> Rho/1

== system eVTOL_System/Dynamics/Variant Subsystem/Sensors/ Baro Simulation ==
  GPS Position : Inport
  Extract Altitude : Selector  InputPortWidth=3  IndexOptions=Index vector (dialog)  Indices=[3]  OutputSizes=1
  Gain1 : Gain  Gain=1/1000
  Gain2 : Gain  Gain=1000
  Lapse Rate Model : aerolibatmos2/ISA Atmosphere Model  useExtended=off  action=Warning  custom=on  viscosityOut=off  g=9.80665  gamma=1.4  R=287.0531  L=0.0065  h_trop=11000  h_strat=20000  rho0=1.225  P0=101325  T0=288.15  h0=0  S=110.4  Tref=273.15  muref=1.716e-5
  Random Number1 : RandomNumber  Variance=10  Seed=10  SampleTime=.1
  Sum1 : Sum  Inputs=|++
  Terminator : Terminator
  Terminator1 : Terminator
  Pressure : Outport
  rho : Outport  Port=2
  wires:
  Lapse Rate Model/2 -> Terminator1/1
  Lapse Rate Model/4 -> rho/1
  Lapse Rate Model/1 -> Terminator/1
  Lapse Rate Model/3 -> Pressure/1
  Sum1/1 -> Gain1/1
  Gain2/1 -> Sum1/1
  Extract Altitude/1 -> Gain2/1
  Gain1/1 -> Lapse Rate Model/1
  GPS Position/1 -> Extract Altitude/1
  Random Number1/1 -> Sum1/2  "Pressure_noise"

== system eVTOL_System/Dynamics/Variant Subsystem/Sensors/Airspeed ==
  In Bus Element : Inport  PortName=States  Element=airspeed
  rho : Inport  Port=2
  Constant : Constant  Value=0.5
  Constant1 : Constant  Value=0
  Max : MinMax  Function=max  Inputs=2
  Product : Product  Inputs=3
  Random Number1 : RandomNumber  Variance=0.1  Seed=545  SampleTime=.1
  Square : Math  Operator=square
  Sum : Sum  Inputs=|++
  Diff Pressure : Outport
  wires:
  Constant/1 -> Product/3
  rho/1 -> Product/2
  Square/1 -> Product/1
  In Bus Element/1 -> Square/1
  Product/1 -> Sum/1
  Random Number1/1 -> Sum/2  "Pressure_noise"
  Max/1 -> Diff Pressure/1
  Sum/1 -> Max/1
  Constant1/1 -> Max/2

== system eVTOL_System/Dynamics/Variant Subsystem/Sensors/Create States Bus for sensors ==
  Ve : Inport
  Xe : Inport  Port=2
  pqr_e : Inport  Port=3
  ypr : Inport  Port=4
  acc_lnav_e : Inport  Port=5
  Airspeed : Inport  Port=6
  AA Filter 2nd Order{,1..7,9..15} (15 alike) : TransferFcn  Numerator=SensorAAFiltNum  Denominator=SensorAAFiltDen
  AA Filter 2nd Order8 : TransferFcn  Numerator=SensorAAFiltNum  Denominator=[1 3.70e+03 6.85e+06]
  Bus Creator : BusCreator  Inputs=X,Y,Z,yaw,pitch,roll,dx,dy,dz,p,q,r,ddx,ddy,ddz,airspeed
  Demux{,1..4} (5 alike) : Demux  Outputs=3
  States : Outport
  wires:
  acc_lnav_e/1 -> Demux/1
  pqr_e/1 -> Demux4/1
  Ve/1 -> Demux3/1
  ypr/1 -> Demux2/1
  Xe/1 -> Demux1/1
  Bus Creator/1 -> States/1
  Demux3/3 -> AA Filter 2nd Order8/1  "dz"
  Demux1/3 -> AA Filter 2nd Order2/1  "Z"
  Demux3/2 -> AA Filter 2nd Order7/1  "dy"
  Demux1/2 -> AA Filter 2nd Order1/1  "Y"
  Demux3/1 -> AA Filter 2nd Order6/1  "dx"
  Demux1/1 -> AA Filter 2nd Order/1  "X"
  Demux/1 -> AA Filter 2nd Order12/1  "ddx"
  Demux4/1 -> AA Filter 2nd Order9/1  "p"
  Demux2/1 -> AA Filter 2nd Order3/1  "yaw"
  Demux/2 -> AA Filter 2nd Order13/1  "ddy"
  Demux2/2 -> AA Filter 2nd Order4/1  "pitch"
  Demux/3 -> AA Filter 2nd Order14/1  "ddz"
  Demux2/3 -> AA Filter 2nd Order5/1  "roll"
  Demux4/2 -> AA Filter 2nd Order10/1  "q"
  Demux4/3 -> AA Filter 2nd Order11/1  "r"
  Airspeed/1 -> AA Filter 2nd Order15/1  "airspeed"
  AA Filter 2nd Order/1 -> Bus Creator/1  "X"
  AA Filter 2nd Order1/1 -> Bus Creator/2  "Y"
  AA Filter 2nd Order2/1 -> Bus Creator/3  "Z"
  AA Filter 2nd Order3/1 -> Bus Creator/4  "yaw"
  AA Filter 2nd Order4/1 -> Bus Creator/5  "pitch"
  AA Filter 2nd Order5/1 -> Bus Creator/6  "roll"
  AA Filter 2nd Order6/1 -> Bus Creator/7  "dx"
  AA Filter 2nd Order7/1 -> Bus Creator/8  "dy"
  AA Filter 2nd Order8/1 -> Bus Creator/9  "dz"
  AA Filter 2nd Order9/1 -> Bus Creator/10  "p"
  AA Filter 2nd Order10/1 -> Bus Creator/11  "q"
  AA Filter 2nd Order11/1 -> Bus Creator/12  "r"
  AA Filter 2nd Order12/1 -> Bus Creator/13  "ddx"
  AA Filter 2nd Order13/1 -> Bus Creator/14  "ddy"
  AA Filter 2nd Order14/1 -> Bus Creator/15  "ddz"
  AA Filter 2nd Order15/1 -> Bus Creator/16  "airspeed"

== system eVTOL_System/Dynamics/Variant Subsystem/Sensors/GNSS//GPS Simulation ==
  States : Inport
  Bus Selector : BusSelector  OutputSignals=dx,dy,dz  OutputAsBus=on
  Bus Selector1 : BusSelector  OutputSignals=X,Y,Z  OutputAsBus=on
  GPS1 : sensorgpslib/GPS  DispRefFrame=NED  PositionInputFormat=Local  ReferenceLocation=[0 0 0]  HorizontalPositionAccuracy=0.01  VerticalPositionAccuracy=0.01  VelocityAccuracy=0.01  DecayFactor=0  SeedDouble=67  SimulateUsing=Code generation
  Reshape1 : Reshape  OutputDimensionality=Row vector (2-D)
  Reshape3 : Reshape  OutputDimensionality=Row vector (2-D)
  Scope : Scope
  Velocity : Outport
  GndSpeed : Outport  Port=2
  Course : Outport  Port=3
  LLA : Outport  Port=4
  wires:
  Reshape3/1 -> GPS1/1
  GPS1/1 -> LLA/1  "lla"
  Bus Selector1/1 -> Reshape3/1
  Bus Selector/1 -> Reshape1/1
  Reshape1/1 -> GPS1/2
  GPS1/2 -> Scope/1, Velocity/1
  States/1 -> Bus Selector/1, Bus Selector1/1
  GPS1/3 -> GndSpeed/1
  GPS1/4 -> Course/1

== system eVTOL_System/Dynamics/Variant Subsystem/Sensors/IMU Simulation ==
  note: Note:
      | we need specific force (accelerometer output) in A-G form, but block gives G-A.
  States : Inport
  Bus Selector1 : BusSelector  OutputSignals=p,q,r  OutputAsBus=on
  Bus Selector2 : BusSelector  OutputSignals=yaw,pitch,roll  OutputAsBus=on
  Bus Selector3 : BusSelector  OutputSignals=ddx,ddy,ddz  OutputAsBus=on
  Coordinate Transformation Conversion : robotcorelib/Coordinate Transformation Conversion  InputRepresentation=Euler Angles  InputEulerSequence=ZYX  ShowTrVecInputPort=on  OutputRepresentation=Rotation Matrix  OutputEulerSequence=ZYX  ShowTrVecOutputPort=on  SimulateUsing=Code generation
  Gain : Gain  Gain=[-1 -1 -1]
  IMU1 : mspsensorlib/IMU  DispRefFrame=NED  TemperaturePort=off  Temperature=25  MagneticFieldPort=off  MagneticFieldNED=[27.5550,-2.4169,-16.0849]  MagneticFieldENU=[ -2.4169, 27.5550, 16.0849 ]  SeedDouble=87254  SimulateUsing=Code generation  AccelParamsMeasurementRange=Inf  AccelParamsResolution=0  AccelParamsConstantBias=[ 0, 0, 0 ]  AccelParamsAxesMisalignment=[ 0, 0, 0 ]  AccelParamsNoiseDensity=0.0003  AccelParamsBiasInstability=[ 0, 0, 0 ]  AccelParamsBiasInstabilityNumerator=fractalcoef().Numerator  AccelParamsBiasInstabilityDenominator=fractalcoef().Denominator  AccelParamsRandomWalk=[ 0, 0, 0 ]  AccelParamsNoiseType=double-sided  AccelParamsTemperatureBias=[ 0, 0, 0 ]  AccelParamsTemperatureScaleFactor=[ 0, 0, 0 ]  GyroParamsMeasurementRange=Inf  GyroParamsResolution=0  GyroParamsConstantBias=[ 0, 0, 0 ]  GyroParamsAxesMisalignment=[ 0, 0, 0 ]  GyroParamsAccelerationBias=0.0001  GyroParamsNoiseDensity=0.0002  GyroParamsBiasInstability=[ 0, 0, 0 ]  GyroParamsBiasInstabilityNumerator=fractalcoef().Numerator  GyroParamsBiasInstabilityDenominator=fractalcoef().Denominator  GyroParamsRandomWalk=[ 0, 0, 0 ]  GyroParamsNoiseType=double-sided  GyroParamsTemperatureBias=[ 0, 0, 0 ]  GyroParamsTemperatureScaleFactor=[ 0, 0, 0 ]  MagParamsMeasurementRange=Inf  MagParamsResolution=0  MagParamsConstantBias=[ 0, 0, 0 ]  MagParamsAxesMisalignment=[ 0, 0, 0 ]  MagParamsNoiseDensity=0.0005  MagParamsBiasInstability=[ 0, 0, 0 ]  MagParamsBiasInstabilityNumerator=fractalcoef().Numerator  MagParamsBiasInstabilityDenominator=fractalcoef().Denominator  MagParamsRandomWalk=[ 0, 0, 0 ]  MagParamsNoiseType=double-sided  MagParamsTemperatureBias=[ 0, 0, 0 ]  MagParamsTemperatureScaleFactor=[ 0, 0, 0 ]
  Reshape : Reshape  OutputDimensionality=Row vector (2-D)
  Reshape2 : Reshape  OutputDimensionality=Row vector (2-D)
  Scope : Scope
  Transpose : Math  Operator=transpose
  Acc : Outport
  Gyro : Outport  Port=2
  Mag : Outport  Port=3
  wires:
  Reshape/1 -> Gain/1
  Bus Selector3/1 -> Reshape/1
  Bus Selector1/1 -> Reshape2/1
  Bus Selector2/1 -> Coordinate Transformation Conversion/1
  Reshape2/1 -> IMU1/2
  States/1 -> Bus Selector1/1, Bus Selector2/1, Bus Selector3/1
  Coordinate Transformation Conversion/1 -> Transpose/1
  IMU1/1 -> Scope/1, Acc/1
  IMU1/3 -> Mag/1
  IMU1/2 -> Gyro/1
  Gain/1 -> IMU1/1
  Transpose/1 -> IMU1/3
